simulink model "RCAM"  (R2024b)
settings: Solver=VariableStepAuto  StartTime=0.0  StopTime=inf  FixedStep=0.0000111111111111111111111111111  RelTol=1e-3
libraries: aerolibfltsims x2, aerolibanim x1, aerolibanimutils x1
settings Model: Creator=AAAR  LastModifiedBy=AAAR

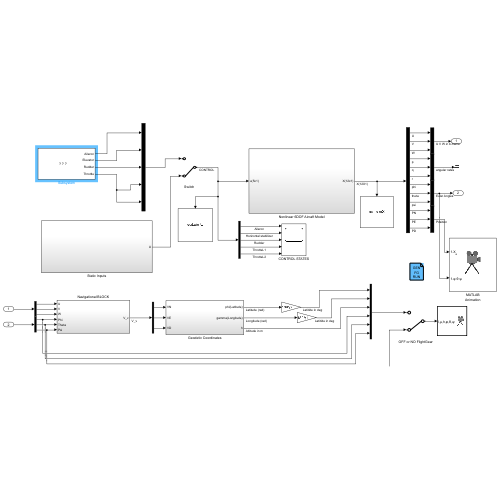
[thumbnail: Simulink's stored preview of the top-level diagram]
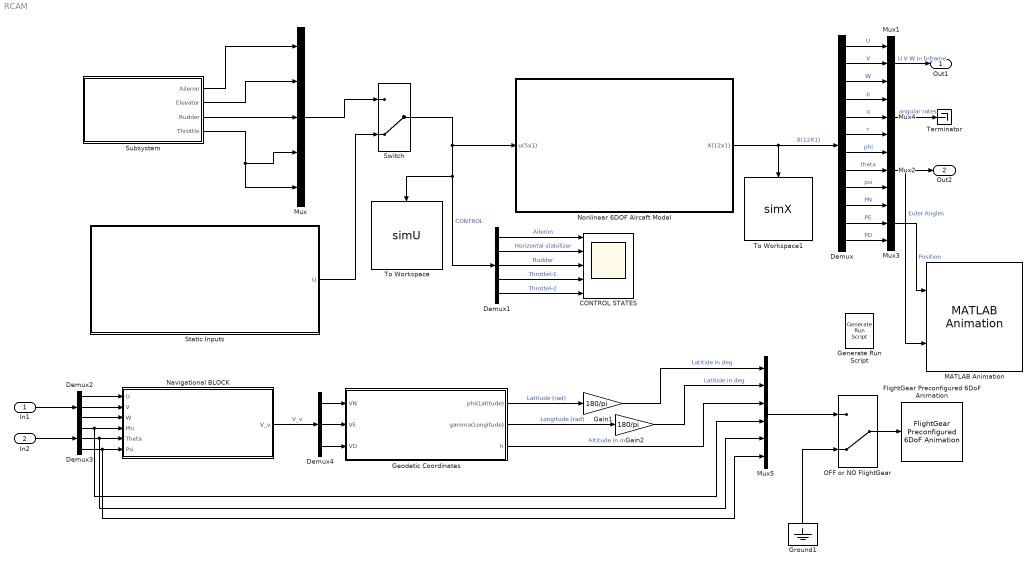
== system RCAM ==
  In1 : Inport
  In2 : Inport  Port=2
  "CONTROL STATES " : Scope  NumInputPorts=5
  Demux : Demux  Outputs=12
  Demux1 : Demux  Outputs=5
  Demux2 : Demux  Outputs=3
  Demux3 : Demux  Outputs=3
  Demux4 : Demux  Outputs=3
  FlightGear Preconfigured 6DoF Animation : aerolibfltsims/FlightGear Preconfigured 6DoF Animation  xFlightGearVersion=v2019.1  DestinationIpAddress=127.0.0.1  DestinationPort=5502  SampleTime=1/30  packetVersion=24
  Gain1 : Gain  Gain=180/pi
  Gain2 : Gain  Gain=180/pi
  Generate Run Script : aerolibfltsims/Generate Run Script  Architecture=Win64  dataFlow=Send  GeometryModelName=c172p  AirportId=KSFO  RunwayId=10L  InitialAltitude=7224  InitialHeading=113  OffsetDistance=4.72  OffsetAzimuth=0  InstallScenery=off  DisableShaders=off  OriginAddress=127.0.0.1  DestinationPort=5502  OriginPort=5505  LocalAddress=127.0.0.1  OutputFileName=runfg.bat  FlightGearBaseDirectory=E:\$ 00 My Data\FlightGear 2020.3
  Geodetic Coordinates : Subsystem
  Ground1 : Ground
  MATLAB Animation : aerolibanim/MATLAB Animation  Tag=Matlab Animation 6 DOF  Vehicles=1  Geometries='pa24-250_orange.ac'  BoundingBoxCoordinates=[-50,50,-50,50,-50,50]  CameraOffset=[-150,-50,0]  CameraViewAngle=3  SampleTime=0.2  FigurePosition=[107,130,634,724]
  Mux : Mux  Inputs=5
  Mux{1..4} (4 alike) : Mux  Inputs=3
  Mux5 : Mux  Inputs=6
  Navigational BLOCK : Subsystem
  Nonlinear 6DOF Aircaft Model : Subsystem
  OFF or NO FlightGear : ManualSwitch  CurrentSetting=0
  Static Inputs : Subsystem
  Subsystem : Subsystem
      mask Display: image('DS4.jpeg');
  Switch : ManualSwitch  CurrentSetting=0
  Terminator : Terminator
  To Workspace : ToWorkspace  VariableName=simU  SaveFormat=Timeseries  SampleTime=-1
  To Workspace1 : ToWorkspace  VariableName=simX  SaveFormat=Timeseries  SampleTime=-1
  Out1 : Outport
  Out2 : Outport  Port=2
  wires:
  Subsystem/1(Aileron) -> Mux/1
  Subsystem/2(Elevator) -> Mux/2
  Subsystem/3(Rudder) -> Mux/3
  Subsystem/4(Throttle) -> Mux/5, Mux/4
  Static Inputs/1(U) -> Switch/2
  Mux/1 -> Switch/1
  Demux1/5 -> "CONTROL STATES "/5  "Throttel-2"
  Demux1/3 -> "CONTROL STATES "/3  "Rudder"
  Demux1/2 -> "CONTROL STATES "/2  "Horizontal stabilizer"
  Demux1/4 -> "CONTROL STATES "/4  "Throttel-1"
  Demux1/1 -> "CONTROL STATES "/1  "Aileron"
  Switch/1 -> Nonlinear 6DOF Aircaft Model/1(u(5x1)), Demux1/1, To Workspace/1  "CONTROL"
  Demux/10 -> Mux3/1  "PN"
  Demux/2 -> Mux1/2  "V"
  Demux/7 -> Mux2/1  "phi"
  Demux/5 -> Mux4/2  "q"
  Demux/11 -> Mux3/2  "PE"
  Demux/4 -> Mux4/1  "p"
  Demux/6 -> Mux4/3  "r"
  Demux/9 -> Mux2/3  "psi"
  Demux/1 -> Mux1/1  "U"
  Demux/12 -> Mux3/3  "PD"
  Demux/3 -> Mux1/3  "W"
  Demux/8 -> Mux2/2  "theta"
  Mux4/1 -> Terminator/1  "angular rates"
  Demux2/1 -> Navigational BLOCK/1(U)
  Demux2/2 -> Navigational BLOCK/2(V)
  Demux2/3 -> Navigational BLOCK/3(W)
  Mux1/1 -> Out1/1  "U V W in b-frame"
  Demux3/1 -> Mux5/4, Navigational BLOCK/4(Phi)
  Demux3/2 -> Mux5/5, Navigational BLOCK/5(Theta)
  Demux3/3 -> Mux5/6, Navigational BLOCK/6(Psi)
  Navigational BLOCK/1(V_v) -> Demux4/1  "V_v"
  Demux4/1 -> Geodetic Coordinates/1(VN)
  Demux4/2 -> Geodetic Coordinates/2(VE)
  Demux4/3 -> Geodetic Coordinates/3(VD)
  Geodetic Coordinates/1(phi(Latitude)) -> Gain1/1  "Latitude (rad)"
  Geodetic Coordinates/2(gamma(Longitude)) -> Gain2/1  "Longitude (rad)"
  Gain1/1 -> Mux5/1  "Latitide in deg"
  Gain2/1 -> Mux5/2  "Latitide in deg"
  Geodetic Coordinates/3(h) -> Mux5/3  "Altitude in m"
  Mux5/1 -> OFF or NO FlightGear/1
  Ground1/1 -> OFF or NO FlightGear/2
  OFF or NO FlightGear/1 -> FlightGear Preconfigured 6DoF Animation/1
  Nonlinear 6DOF Aircaft Model/1(X(12x1)) -> Demux/1, To Workspace1/1  "X(12X1)"
  Mux3/1 -> MATLAB Animation/1  "Position"
  In1/1 -> Demux2/1
  Mux2/1 -> Out2/1, MATLAB Animation/2  "Euler Angles"
  In2/1 -> Demux3/1

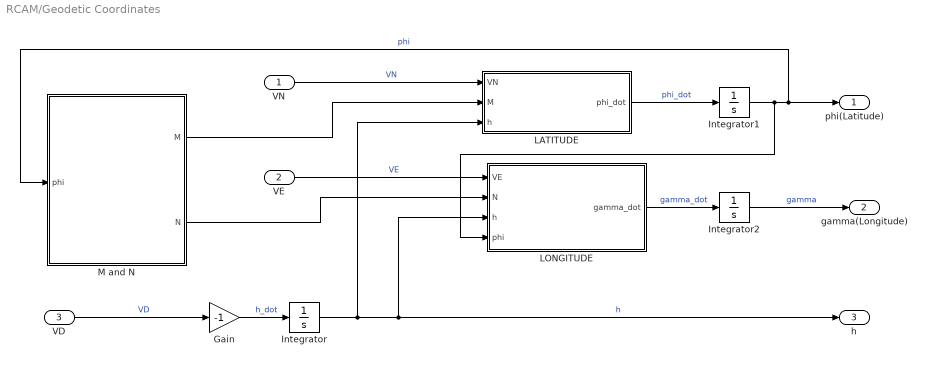
== system RCAM/Geodetic Coordinates ==
  VN : Inport
  VE : Inport  Port=2
  VD : Inport  Port=3
  Gain : Gain  Gain=-1
  Integrator : Integrator  InitialCondition=150
  Integrator1 : Integrator  InitialCondition=0.22181
  Integrator2 : Integrator  InitialCondition=1.356068
  LATITUDE : MATLAB Function  TreatAsAtomicUnit=on
  LONGITUDE : MATLAB Function  TreatAsAtomicUnit=on
  M and N : Subsystem
  phi(Latitude) : Outport
  gamma(Longitude) : Outport  Port=2
  h : Outport  Port=3
  wires:
  VD/1 -> Gain/1  "VD"
  Gain/1 -> Integrator/1  "h_dot"
  Integrator/1 -> LATITUDE/3(h), LONGITUDE/3(h), h/1  "h"
  M and N/1(M) -> LATITUDE/2(M)
  M and N/2(N) -> LONGITUDE/2(N)
  LATITUDE/1(phi_dot) -> Integrator1/1  "phi_dot"
  Integrator1/1 -> LONGITUDE/4(phi), M and N/1(phi), phi(Latitude)/1  "phi"
  VE/1 -> LONGITUDE/1(VE)  "VE"
  VN/1 -> LATITUDE/1(VN)  "VN"
  LONGITUDE/1(gamma_dot) -> Integrator2/1  "gamma_dot"
  Integrator2/1 -> gamma(Longitude)/1  "gamma"

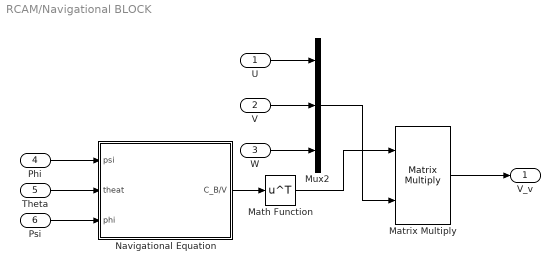
== system RCAM/Navigational BLOCK ==
  U : Inport
  V : Inport  Port=2
  W : Inport  Port=3
  Phi : Inport  Port=4
  Theta : Inport  Port=5
  Psi : Inport  Port=6
  Math Function : Math  Operator=transpose
  Matrix Multiply : Product  Multiplication=Matrix(*)
  Mux2 : Mux  Inputs=3
  Navigational Equation : Subsystem
  V_v : Outport
  wires:
  Mux2/1 -> Matrix Multiply/2
  Math Function/1 -> Matrix Multiply/1
  Phi/1 -> Navigational Equation/1(psi)
  U/1 -> Mux2/1
  Theta/1 -> Navigational Equation/2(theat)
  Matrix Multiply/1 -> V_v/1
  Navigational Equation/1(C_B/V) -> Math Function/1
  W/1 -> Mux2/3
  Psi/1 -> Navigational Equation/3(phi)
  V/1 -> Mux2/2

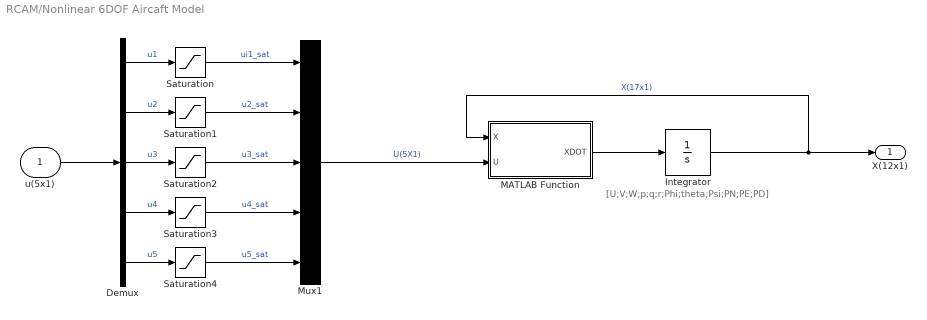
== system RCAM/Nonlinear 6DOF Aircaft Model ==
  note: [U;V;W;p;q;r;Phi;theta;Psi;PN;PE;PD]
  u(5x1) : Inport
  Demux : Demux  Outputs=5
  Integrator : Integrator  InitialCondition=|
      | [84.9905; 0;
      |  1.2713;
      | 0; 0; 0; 0; 0.1; 0; 0; 0.0149; 0]
  MATLAB Function : MATLAB Function  TreatAsAtomicUnit=on
  Mux1 : Mux  Inputs=5
  Saturation : Saturate  UpperLimit=25*(pi/180)  LowerLimit=-15*(pi/180)
  Saturation1 : Saturate  UpperLimit=10*(pi/180)  LowerLimit=-25*(pi/180)
  Saturation2 : Saturate  UpperLimit=30*(pi/180)  LowerLimit=-30*(pi/180)
  Saturation3 : Saturate  UpperLimit=10*(pi/180)  LowerLimit=0.5*(pi/180)
  Saturation4 : Saturate  UpperLimit=10*(pi/180)  LowerLimit=0.5*(pi/180)
  X(12x1) : Outport
  wires:
  Demux/2 -> Saturation1/1  "u2"
  Demux/3 -> Saturation2/1  "u3"
  Demux/4 -> Saturation3/1  "u4"
  MATLAB Function/1(XDOT) -> Integrator/1
  Demux/5 -> Saturation4/1  "u5"
  Saturation3/1 -> Mux1/4  "u4_sat"
  Integrator/1 -> MATLAB Function/1(X), X(12x1)/1  "X(17x1)"
  Saturation1/1 -> Mux1/2  "u2_sat"
  Demux/1 -> Saturation/1  "u1"
  Saturation/1 -> Mux1/1  "ui1_sat"
  Saturation2/1 -> Mux1/3  "u3_sat"
  Mux1/1 -> MATLAB Function/2(U)  "U(5X1)"
  u(5x1)/1 -> Demux/1
  Saturation4/1 -> Mux1/5  "u5_sat"

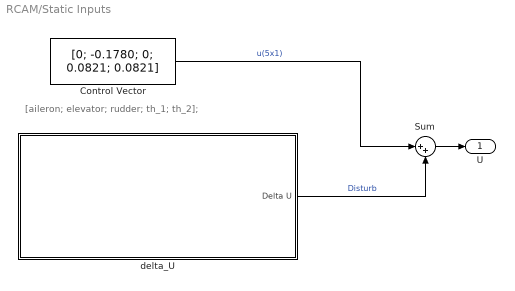
== system RCAM/Static Inputs ==
  note: [aileron; elevator; rudder; th_1; th_2];
  Control Vector : Constant  Value=[0; -0.1780; 0; 0.0821; 0.0821]
  Sum : Sum  Inputs=|++
  delta_U : Subsystem
  U : Outport
  wires:
  delta_U/1(Delta U) -> Sum/2  "Disturb"
  Control Vector/1 -> Sum/1  "u(5x1)"
  Sum/1 -> U/1

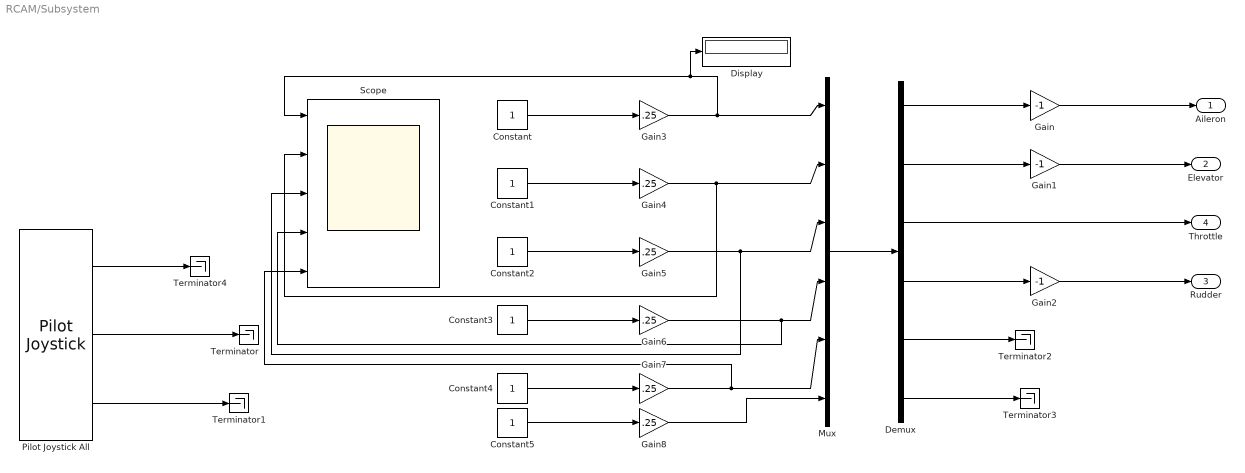
== system RCAM/Subsystem ==
  Constant{,1..5} (6 alike) : Constant
      Constant settings: OpenFcn=set(gcbh,'Value',num2str(double(input('Press a key: ','8'))));
      Constant1 settings: OpenFcn=set(gcbh,'Value',num2str(double(input('Press a key: ','s'))));
      Constant2 settings: OpenFcn=set(gcbh,'Value',num2str(double(input('Press a key: ','s'))));
      Constant3 settings: OpenFcn=set(gcbh,'Value',num2str(double(input('Press a key: ','s'))));
      Constant4 settings: OpenFcn=set(gcbh,'Value',num2str(double(input('Press a key: ','s'))));
      Constant5 settings: OpenFcn=set(gcbh,'Value',num2str(double(input('Press a key: ','s'))));
  Demux : Demux  Outputs=6
  Display : Display
  Gain : Gain  Gain=-1
  Gain1 : Gain  Gain=-1
  Gain2 : Gain  Gain=-1
  Gain{3..8} (6 alike) : Gain  Gain=.25
  Mux : Mux  Inputs=6
  Pilot Joystick All : aerolibanimutils/Pilot Joystick  JoystickID=None  OutputConfiguration=AllOutputs  SampleTime=1/30
  Scope : Scope  NumInputPorts=5
  Terminator{,1..4} (5 alike) : Terminator
  Aileron : Outport
  Elevator : Outport  Port=2
  Rudder : Outport  Port=3
  Throttle : Outport  Port=4
  wires:
  Demux/6 -> Terminator3/1
  Gain2/1 -> Rudder/1
  Pilot Joystick All/2 -> Terminator/1
  Gain/1 -> Aileron/1
  Gain1/1 -> Elevator/1
  Demux/1 -> Gain/1
  Demux/2 -> Gain1/1
  Demux/4 -> Gain2/1
  Demux/3 -> Throttle/1
  Demux/5 -> Terminator2/1
  Pilot Joystick All/3 -> Terminator1/1
  Constant/1 -> Gain3/1
  Pilot Joystick All/1 -> Terminator4/1
  Mux/1 -> Demux/1
  Gain4/1 -> Scope/2, Mux/2
  Constant1/1 -> Gain4/1
  Constant2/1 -> Gain5/1
  Constant3/1 -> Gain6/1
  Constant4/1 -> Gain7/1
  Gain7/1 -> Scope/5, Mux/5
  Gain6/1 -> Scope/4, Mux/4
  Gain5/1 -> Scope/3, Mux/3
  Constant5/1 -> Gain8/1
  Gain8/1 -> Mux/6
  Gain3/1 -> Display/1, Scope/1, Mux/1

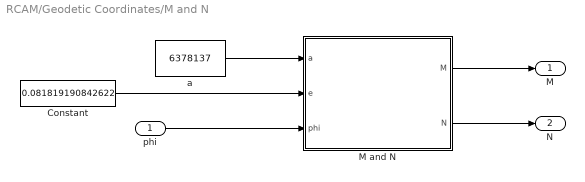
== system RCAM/Geodetic Coordinates/M and N ==
  phi : Inport
  Constant : Constant  Value=0.081819190842622
  M and N : MATLAB Function  TreatAsAtomicUnit=on
  a : Constant  Value=6378137
  M : Outport
  N : Outport  Port=2
  wires:
  Constant/1 -> M and N/2(e)
  phi/1 -> M and N/3(phi)
  M and N/1(M) -> M/1
  a/1 -> M and N/1(a)
  M and N/2(N) -> N/1

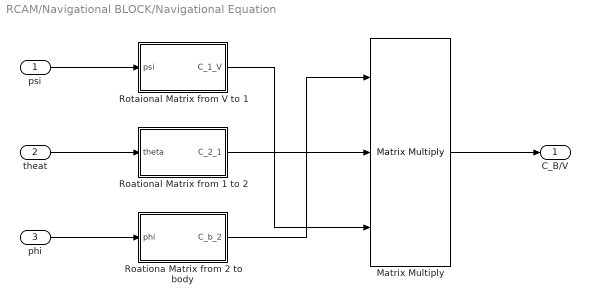
== system RCAM/Navigational BLOCK/Navigational Equation ==
  psi : Inport
  theat : Inport  Port=2
  phi : Inport  Port=3
  Matrix Multiply : Product  Inputs=3  Multiplication=Matrix(*)
  Roationa Matrix from 2 to body : MATLAB Function  TreatAsAtomicUnit=on
  Roational Matrix from 1 to 2 : MATLAB Function  TreatAsAtomicUnit=on
  Rotaional Matrix from V to 1 : MATLAB Function  TreatAsAtomicUnit=on
  C_B/V : Outport
  wires:
  Matrix Multiply/1 -> C_B/V/1
  Rotaional Matrix from V to 1/1(C_1_V) -> Matrix Multiply/3
  Roational Matrix from 1 to 2/1(C_2_1) -> Matrix Multiply/2
  Roationa Matrix from 2 to body/1(C_b_2) -> Matrix Multiply/1
  phi/1 -> Roationa Matrix from 2 to body/1(phi)
  theat/1 -> Roational Matrix from 1 to 2/1(theta)
  psi/1 -> Rotaional Matrix from V to 1/1(psi)

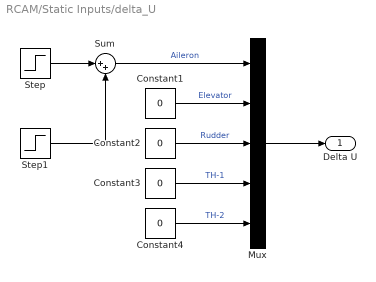
== system RCAM/Static Inputs/delta_U ==
  Constant{1..4} (4 alike) : Constant  Value=0
  Mux : Mux  Inputs=5
  Step : Step  Time=15  After=10*(pi/180)  SampleTime=0
  Step1 : Step  Time=15+5  After=-10*(pi/180)  SampleTime=0
  Sum : Sum  Inputs=|++
  Delta U : Outport
  wires:
  Mux/1 -> Delta U/1
  Constant4/1 -> Mux/5  "TH-2"
  Constant2/1 -> Mux/3  "Rudder"
  Constant3/1 -> Mux/4  "TH-1"
  Constant1/1 -> Mux/2  "Elevator"
  Sum/1 -> Mux/1  "Aileron"
  Step/1 -> Sum/1
  Step1/1 -> Sum/2

== matlab function RCAM/Navigational BLOCK/Navigational Equation/Roational Matrix from 1 to 2 ==
  data: theta input; C_2_1 output
function C_2_1 = fcn(theta)

% Roational Matrix From the 1 frame to 2 frame

C_2_1=[cos(theta) 0 -sin(theta); 0 1 0; sin(theta) 0 cos(theta)];

end

== matlab function RCAM/Nonlinear 6DOF Aircaft Model/MATLAB Function ==
  data: X input; XDOT output; U input
function XDOT  = RCAM_model(X,U)

%----------------STATE AMD CONTROL VECTOR---------------------
%Extract state vector
x1 = X(1); %u
x2 = X(2); %v
x3 = X(3); %w
x4 = X(4); %p
x5 = X(5); %q
x6 = X(6); %r
x7 = X(7); %phi
x8 = X(8); %theta
x9 = X(9); %psi

u1 = U(1); %d_A (aileron)
u2 = U(2); %d_T (stabilizer)
u3 = U(3); %d_R (rudder)
u4 = U(4); %d_th1 (throttle 1)
u5 = U(5); %d_th2 (throttle 2)

%-------------------------CONSTANTS---------------------
%Nominal vehicle constants
m = 120000;                % Aircraft total mass (kg)
%NOTE: We will define Ib and invIb later

cbar = 6.6;                % Mean Aerodynamic Chord (m)
lt = 24.8;                 % Distance by AC of tail and body (m)
S=260;                     % Wing planform area (m^2)
St=64;                     % Tail planform area (m^2)

Xcg=0.23*cbar;             % X Position of cg in Fm (m)
Ycg=0;                     % Y Position of cg in Fm (m)
Zcg=0.10*cbar;             % Z Position of cg in Fm (m)

Xac=0.19*cbar;             % X position of aerodynamic center in Fm (m)
Yac=0;                     % Y position of aerodynamic center in Fm (m)
Zac=0;                     % Z position of aerodynamic center in Fm (m)

% Engine Constants
Xapt1=0;                   % X position of engine 1 force in Fm (m)
Yapt1=-7.94;               % Y position of engine 1 force in Fm (m)
Zapt1=-1.9;                % Z position of engine 1 force in Fm (m)

Xapt2=0;                   % X position of engine 2 force in Fm (m)
Yapt2=7.94;                % Y position of engine 2 force in Fm (m)
Zapt2=-1.9;                % Z position of engine 2 force in Fm (m)

% Other constants
rho=1.225;                 % Air density in (kg/m^3)
g=9.81;                    % Acceleration due to gravity (m/s^2)
depsda=0.25;               % Change in downwash w.r.t alpha (rad/rad)
alpha_L0=-11.5*(pi/180);   % Zero lift angle of attack (rad)
n=5.5;                     % Slope of linear region of lift slope
a3=-768.5;                 % coefficient of alpha^3
a2=609.2;                  % coefficient of alpha^2
a1=-155.2;                 % coefficient of alpha^1
a0=-15.212;                % coefficient of alpha^0 (Different from RCAM Model)
alpha_switch=14.5*(pi/180); % alpha value lift slope goes from linear to non-linear

%--------------------CONTROL SATURATION---------------------
% These control saturation are defined in the Simulink Model. Thus the code is commented
% Note that these can alternatively be enforced in simulink

% u1min=-15*(pi/180);
% u1max=25*(pi/180);
% 
% u2min=-25*(pi/180);
% u2max=10*(pi/180);
% 
% u3min=-30*(pi/180);
% u3max=30*(pi/180);
% 
% u4min=0.5*(pi/180);
% u4max=10*(pi/180);
% 
% u5min=0.5*(pi/180);
% u5max=10*(pi/180);
% 
% if(u1>u1max)
%     u1=u1max;
% elseif(u1<u1min)
%     u1=u1min;
% end
% 
% if(u2>u2max)
%     u2=u2max;
% elseif(u2<u2min)
%     u2=u2min;
% end
% 
% if(u3>u3max)
%     u3=u3max;
% elseif(u3<u3min)
%     u3=u3min;
% end
% 
% if(u4>u4max)
%     u4=u1max;
% elseif(u4<u4min)
%     u4=u4min;
% end
% 
% if(u5>u5max)
%     u5=u5max;
% elseif(u5<u5min)
%     u5=u5min;
% end

%---------------------INTERMEDIATE VARIABLES----------------------
% calculate the airspeed
Va=sqrt(x1^2+x2^2+x3^2);

%claculate the alph and beta
alpha=atan2(x3,x1);
beta=asin(x2/Va);

%claculation of the dynamic pressure
Q=0.5*rho*Va^2;

%Also define the vectors wbe_b and V_b
wbe_b=[x4;x5;x6];
V_b=[x1;x2;x3];

%--NON DIMENSIONAL AERODYNAMIC FORCES COEFFICIENTS IN THE STABILITY FRAME--
% Calculate the CL_wb

if alpha<=alpha_switch

      CL_wb=n*(alpha-alpha_L0);
else
      CL_wb=a3*alpha^3+a2*alpha^2+a1*alpha+a0;
end

%Claculate CL_t

epsilon=depsda*(alpha-alpha_L0);
alpha_t=alpha-epsilon+u2+1.3*x5*lt/Va;
CL_t=3.1*(St/S)*alpha_t;

% claculation of the Total lift force
CL=CL_wb+CL_t;

% Total drag force (Neglecting the tail)
CD=0.13+0.07*(5.5*alpha+0.654)^2;

% Calculate the side force
CY=-1.6*beta+0.24*u3;

%--------------------DIMENSIONAL AERDOYNAMIC FORCES-----------------------
% calculate the actual dimensional forces. These are in F_s (Stability axis)

FA_s=[-CD*Q*S;CY*Q*S;-CL*Q*S];

%----------Rotating the forces from the stability frame to body frame------
% Rotate these forces to F_b (Body axis)
C_bs=[cos(alpha) 0 -sin(alpha);0 1 0;sin(alpha) 0 cos(alpha)];

FA_b=C_bs*FA_s;

%--NON-DIMENSIOANL AERODYNAMIC MOMENT COEFFICIENT ABOUT THE AC IN THE BODY FRAME--
%Calculate the moments in Fb.  Define eta,dCMdx and dCMdu

eta11=-1.4*beta;
eta21=-0.59-(3.1*(St*lt)/(S*cbar))*(alpha-epsilon);
eta31=(1-alpha*(180/(15*pi)))*beta;


eta=[eta11;eta21;eta31];

dCMdx=(cbar/Va)*[-11 0 5;0 (-4.03*(St*lt^2)/(S*cbar^2)) 0;1.7 0 -11.5]; % needed correcction

dCMdu=[-0.6 0 0.22;0 (-3.1*(St*lt)/(S*cbar)) 0;0 0 -0.63];

% Now calculate CM=[cl;cm;cn] about aerodynamic center in Fb
CMac_b=eta+dCMdx*wbe_b+dCMdu*[u1;u2;u3];

%------------AERODYNAMIC MOMENT ABOUT AC IN THE BODY FRAME---------------
%Normalize to an aerodynamic moments
MAac_b=CMac_b*Q*S*cbar;

%--------------AERODYNAMIC MOMENT ABOUT CG IN BODY FRAME-------------
%Transfer moment to CG
rcg_b=[Xcg;Ycg;Zcg];
rac_b=[Xac;Yac;Zac];

MAcg_b=MAac_b+cross(FA_b,rcg_b-rac_b);

%-------------------------PROPULSION EFFECTS----------------------------
% First, calculate the thrust of each engine

F1=u4*m*g;
F2=u5*m*g;

%Assuming that the engine thrust is aligned with the Fb, we have

FE1_b=[F1;0;0];
FE2_b=[F2;0;0];

FE_b=FE1_b+FE2_b;

%Now the engine moment due to offset of engine thrust from cog

mew1=[Xcg-Xapt1;Yapt1-Ycg;Zcg-Zapt1];
mew2=[Xcg-Xapt2;Yapt2-Ycg;Zcg-Zapt2];

MEcg1_b=cross(mew1,FE1_b);
MEcg2_b=cross(mew2,FE2_b);

MEcg_b=MEcg1_b+MEcg2_b;

%--------------------------GRAVITY EFFECTS----------------------------
% Cosidering the FLAT EARTH EQUATIONS
% Calculate the gravitational forces in the body frame. This causes no moments abot the CG
g_b=[-g*sin(x8);g*cos(x8)*sin(x7);g*cos(x8)*cos(x7)];

Fg_b=m*g_b;

%-------------------EXPLICIT FIRST ORDER FORM-------------------------
%Inertia matrix
Ib=m*[40.07 0 -2.0923;0 64 0;-2.0923 0 99.92];

% Inverse of the inertia matrix
invIb=(1/m)*[0.0249836 0 0.000523151;0 0.015625 0;0.000523215 0 0.010019];

% From F_b ( all the forces in Fb ) and calculate the udot, vdot,wdot
F_b=Fg_b+FE_b+FA_b;
x1to3dot=(1/m)*F_b-cross(wbe_b,V_b);

%From Mcg_b (all the moments about the cog in Fb) and calculate pdot,qdpt,rdoot
Mcg_b=MAcg_b+MEcg_b;
x4to6dot=invIb*(Mcg_b-cross(wbe_b,Ib*wbe_b));

% Calculation of the phidot,thetadot,psidot
H_pi=[1 sin(x7)*tan(x8) cos(x7)*tan(x8);0 cos(x7) -sin(x7);0 sin(x7)/cos(x8) cos(x7)/cos(x8)];
x7to9dot=H_pi*wbe_b;

%-----------------------------NAVIGATION EQUATION----------------------
% Rotational Matrix from the 1 frame to 2 frame
C1v=[cos(x9) sin(x9) 0;
    -sin(x9) cos(x9) 0;
    0 0 1];

% Rotational Matrix from the 1 frame to 2 frame
C21=[cos(x8) 0 -sin(x8);
    0 1 0;
    sin(x8) 0 cos(x8)];

% Rotational Matrix from the 1 frame to 2 frame
Cb2=[1 0 0;
    0 sin(x7) cos(x7);
    0 -sin(x7) cos(x7)];

% Implimenting the Navigational Equation
Cbv=Cb2*C21*C1v;
Cvb=Cbv';
x10to12dot=Cvb*V_b;

%-------------------EXPLICIT FIRST ORDER FORM-------------------------
XDOT=[x1to3dot;
    x4to6dot;
    x7to9dot;
    x10to12dot;
    ];

== matlab function RCAM/Navigational BLOCK/Navigational Equation/Roationa Matrix from 2 to body ==
  data: phi input; C_b_2 output
function C_b_2 = fcn(phi)

% Roational Matrix from the 2 frame to body frame
C_b_2=[1 0 0; 0 cos(phi) sin(phi); 0 -sin(phi) cos(phi)];
end

== matlab function RCAM/Navigational BLOCK/Navigational Equation/Rotaional Matrix from V to 1 ==
  data: psi input; C_1_V output
function C_1_V = fcn(psi)

% Calculating the Rotaional Matrix  from the NED to 1 frame

C_1_V=[cos(psi) sin(psi) 0; -sin(psi) cos(psi) 0; 0 0 1];

end

== matlab function RCAM/Geodetic Coordinates/LATITUDE ==
  data: VN input; phi_dot output; M input; h input
function phi_dot =Latitude_Rate(VN,M,h)
% Calculating the Rate of change of Latitude

phi_dot=VN/(M+h);
end

== matlab function RCAM/Geodetic Coordinates/LONGITUDE ==
  data: VE input; gamma_dot output; N input; h input; phi input
function gamma_dot =Longitude_Rate(VE,N,h,phi)

% Calculating the Rate of change of the Longitude

gamma_dot=VE/((N+h)*cos(phi));
end

== matlab function RCAM/Geodetic Coordinates/M and N/M and N ==
  data: a input; M output; e input; phi input; N output
function[M,N]=M_N(a,e,phi)

M=(a*(1-e*2)/(1-(e^2)*sin(phi))^3/2);  % Meridian Radius of Curvature

N=a/(1-(e^2)*(sin(phi)^2))^3/2;        % Prime verical radius of curvature

end
